simulink model "VSCHVDCunitblackstart"  (R2025b)
settings: Solver=VariableStepAuto  StartTime=0  StopTime=25  FixedStep=5e-5  RelTol=1e-3
PreLoadFcn:
  | HVDCParameters;
  | BlackStartMMCParameters;
undefined symbols (not defined in the file): DiscIntNeverNeededParam, FRated, frt, gGFM, grid, Lbase, Lr, Lt, lvrt, mGFM, mpptOmega, mpptWindSpeed, Nm, pmsm, PRated, Rc, rpir, Rr, Rt, time, Tpir, Ts, Vbase, Vdcs0, VRated, Vt2, windController, windTurbine, Zbase
libraries: fl_lib x47, ee_lib x41, nesl_utility x33, eeGeneralControl x13, eeTransforms x12, slpidlib x8, eeSinusoidalMeasurementV2 x4, simulink x2, eeSinusoidalMeasurement x1, eeStairGenerator x1
(part 3 of 5)

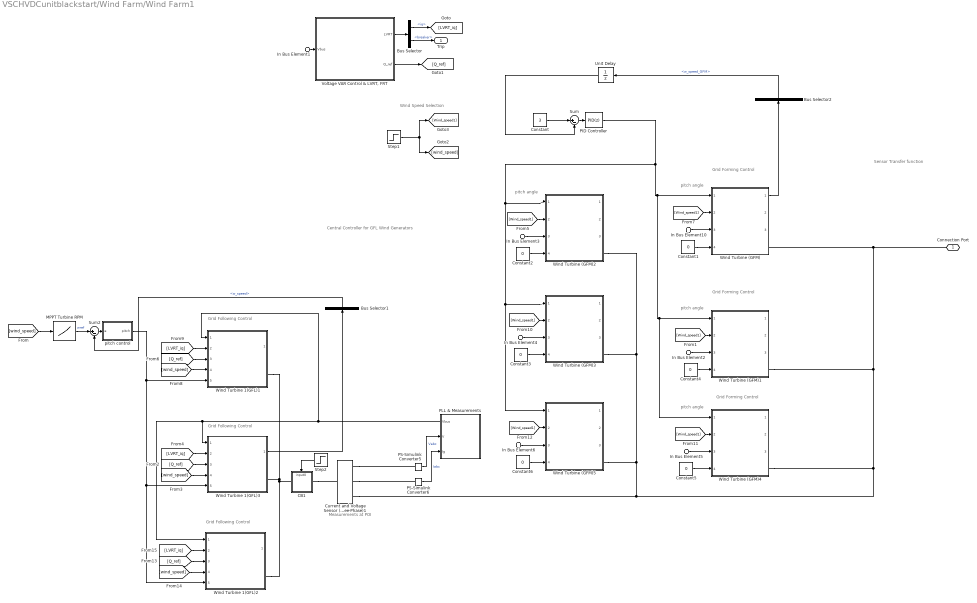
== system VSCHVDCunitblackstart/Wind Farm/Wind Farm1 ==
  note: Central Controller for GFL Wind Generators
  note: Wind Speed Selection
  note: Sensor Transfer function
  note: pitch angle
  note: Grid Forming Control
  note: Grid Forming Control
  note: pitch angle
  note: Grid Forming Control
  note: Measurements at POI
  note: pitch angle
  note: pitch angle
  note: Grid Following Control
  note: Grid Following Control
  note: Grid Following Control
  In Bus Element{1..6,10} (7 alike) : Inport  PortName=us
  Bus Selector : BusSelector  OutputSignals=iq,breaker
  Bus Selector1 : BusSelector  OutputSignals=w_speed
  Bus Selector2 : BusSelector  OutputSignals=w_speed_GFM
  CB1 : Subsystem
      settings: PortSchema="{\"entries\":[{\"content\":{\"sides\":[{\"content\":{\"connectorIds\":[\"LConn1\"]},\"type\":\"ConnectorPlacement.EquallySpacedRectSide\",\"uuid\":\"67c0f727-7c15-41c9-98df-b3c7d57498ed\"},{\"content\":{\"connectorIds\":[\"RConn1\"],\"side\":\"RIGHT\"},\"type\":\"ConnectorPlacement.EquallySpacedRectSide\",\"uuid\":\"7fc39429-ba61-416d-b42b-93e81eb2f426\"},{\"content\":{\"side\":\"TOP\"},\"type\":\"ConnectorPlacement.EquallySpacedRectSide\",\"uuid\":\"c6dd9263-b57a-4cff-a218-af99f2798f29\"},{\"content\":{\"connectorIds\":[\"In1\"],\"side\":\"BOTTOM\"},\"type\":\"ConnectorPlacement.EquallySpacedRectSide\",\"uuid\":\"e2a2ba44-d59d-4e27-adf1-3f94e828ca78\"}]},\"type\":\"ConnectorPlacement.EquallySpacedConnector\",\"uuid\":\"b349a99b-c902-4df9-9c99-34841afb28dd\"}],\"packageUris\":[\"http://schema.mathworks.com/mf0/Connector/R2020b\"],\"version\":\"1.0\"}"
  Constant : Constant  Value=3
  Constant{1..6} (6 alike) : Constant  Value=0
  Current and Voltage Sensor (Three-Phase)1 : ee_lib/Sensors & Transducers/Current and Voltage Sensor (Three-Phase)  vMeasurementType=ee.enum.vmeasurement.lg  outputUnit=ee.enum.unit.pu  SRated=base.mVA A*V  VRated=base.kV V  I_specify=off  I_priority=None  I=[0, 0, 0] A  I_nominal_specify=off  I_nominal_value=1  I_nominal_unit=A  V_specify=off  V_priority=None  V=[0, 0, 0] V  V_nominal_specify=off  V_nominal_value=1  V_nominal_unit=V
      settings: InternalSimscapePortConfiguration="{\"Bottom\":[],\"Left\":[{\"id\":\"N1\",\"label\":\"~1\",\"type\":\"foundation.electrical.three_phase\"}],\"Right\":[{\"id\":\"V_output\",\"label\":\"V\",\"type\":\"output\"},{\"id\":\"I_output\",\"label\":\"I\",\"type\":\"output\"},{\"id\":\"N2\",\"label\":\"~2\",\"type\":\"foundation.electrical.three_phase\"}],\"Top\":[]}"
  MPPT Turbine RPM : Lookup_n-D  NumberOfTableDimensions=1  BreakpointsForDimension1=mpptWindSpeed  Table=mpptOmega  InternalRulePriority=Speed  RndMeth=Simplest
  PID Controller : slpidlib/PID Controller  Controller=PID  Form=Parallel  TimeDomain=Discrete-time  UseExternalTs=off  SampleTime=-1  IntegratorMethod=Forward Euler  FilterMethod=Forward Euler  ControllerParametersSource=internal  P=-0.5  I=-1  UseKiTs=off  D=0  UseExternalDerivativeSource=off  N=100  UseFilter=on  TunerSelectOption=Transfer Function Based (PID Tuner App)  InitialConditionSource=internal  InitialConditionForIntegrator=0  InitialConditionForFilter=0  DifferentiatorICPrevScaledInput=0  ExternalReset=none  TrackingMode=off  Kt=1  LimitOutput=off  SatLimitsSource=internal  UpperSaturationLimit=20  LowerSaturationLimit=-20  LinearizeAsGain=on  AntiWindupMode=back-calculation  Kb=1  LimitIntegrator=off  UpperIntegratorSaturationLimit=inf  LowerIntegratorSaturationLimit=-inf  POutMin=[]  POutMax=[]  IOutMin=[]  IOutMax=[]  DOutMin=[]  DOutMax=[]  NOutMin=[]  NOutMax=[]  SumOutMin=[]  SumOutMax=[]  SaturationOutMin=[]  SaturationOutMax=[]  PParamMin=[]  PParamMax=[]  IParamMin=[]  IParamMax=[]  DParamMin=[]  DParamMax=[]  NParamMin=[]  NParamMax=[]  KbParamMin=[]  KbParamMax=[]  KtParamMin=[]  KtParamMax=[]  KbOutMin=[]  KbOutMax=[]  KtOutMin=[]  KtOutMax=[]  IntegratorOutMin=[]  IntegratorOutMax=[]  FilterOutMin=[]  FilterOutMax=[]  SumI1OutMin=[]  SumI1OutMax=[]  SumI2OutMin=[]  SumI2OutMax=[]  SumI3OutMin=[]  SumI3OutMax=[]  SumI4OutMin=[]  SumI4OutMax=[]  SumDOutMin=[]  SumDOutMax=[]  DifferentiatorOutMin=[]  DifferentiatorOutMax=[]  FilterDiffOutCoefMin=[]  FilterDiffOutCoefMax=[]  ReciprocalOutMin=[]  ReciprocalOutMax=[]  SumDenOutMin=[]  SumDenOutMax=[]  SumNumOutMin=[]  SumNumOutMax=[]  DivideOutMin=[]  DivideOutMax=[]  UdiffTsProdOutMin=[]  UdiffTsProdOutMax=[]  NTsProdOutMin=[]  NTsProdOutMax=[]  UintegralTsProdOutMin=[]  UintegralTsProdOutMax=[]  UngainTsProdOutMin=[]  UngainTsProdOutMax=[]  ClampingZeroOutDataTypeStr=Inherit: Inherit via back propagation  ClampingZeroOutMin=[]  ClampingZeroOutMax=[]  FilterDenConstantOutDataTypeStr=Inherit: Inherit via back propagation  FilterDenConstantOutMin=[]  FilterDenConstantOutMax=[]  PCopyOutDataTypeStr=Inherit: Inherit via back propagation  PCopyOutMin=[]  PCopyOutMax=[]  NCopyOutDataTypeStr=Inherit: Inherit via back propagation  NCopyOutMin=[]  NCopyOutMax=[]  IntegratorContinuousStateAttributes=''  IntegratorStateMustResolveToSignalObject=off  IntegratorRTWStateStorageClass=Auto  FilterContinuousStateAttributes=''  FilterStateMustResolveToSignalObject=off  FilterRTWStateStorageClass=Auto  ParallelPVariant=InternalParameters  IdealPVariant=Disabled  IVariant=InternalParameters  DVariant=InternalParameters  IntegratorVariant=Discrete  SatVariant=Disabled  AWVariant=Passthrough  PCopyVariant=Disabled  TRVariant=Disabled  FdbkBlocksVariant=Forward  IdealPFdbkVariant=Disabled  SatFdbkVariant=Disabled  DerivativeFilterVariant=ForwardEulerFilter  NVariant=InternalParameters  NCopyVariant=Disabled  FilterICVariant=InternalICsFilter  IntegratorICVariant=InternalICs  ExternalResetVariant=Disabled  TRSumVariant=Passthrough  SumFdbkVariant=Disabled  SumVariant=Sum_PID  TsampFilterVariant=InternalTs  TsampNgainVariant=Passthrough  TsampIntegralVariant=Disabled_SignalSpec  ExternalSaturationOutDataTypeStr=Inherit: Same as second input  DerivativeSourceVariant=ErrorSignal  PreIntVariant=InternalPreInt
  PLL & Measurements : Subsystem
      settings: PortSchema="{\"entries\":[{\"content\":{\"sides\":[{\"content\":{\"connectorIds\":[\"Out1\",\"In1\",\"In2\"]},\"type\":\"ConnectorPlacement.EquallySpacedRectSide\",\"uuid\":\"76485780-20fe-4fcf-8224-69648da6ed2a\"},{\"content\":{\"side\":\"RIGHT\"},\"type\":\"ConnectorPlacement.EquallySpacedRectSide\",\"uuid\":\"f19a6390-e634-42c7-8d46-4cd80cbab182\"},{\"content\":{\"side\":\"TOP\"},\"type\":\"ConnectorPlacement.EquallySpacedRectSide\",\"uuid\":\"87682f72-1844-428e-be70-ad7ca3191ee3\"}]},\"type\":\"ConnectorPlacement.EquallySpacedConnector\",\"uuid\":\"f2136b07-48ec-402b-adb3-18c0bac2157c\"}],\"packageUris\":[\"http://schema.mathworks.com/mf0/Connector/R2020b\"],\"version\":\"1.0\"}"
      mask Display: image('measurements.png'); % Use "Edit Image" on toolstrip to change.
  PS-Simulink Converter5 : nesl_utility/PS-Simulink Converter  PhysicalDomain=network_engine_domain  SubClassName=ps_output  LeftPortType=input  RightPortType=output  PseudoPeriodic=off  Frequencies=[]  VectorFormat=inherit  Unit=inherit  AffineConversion=off
  PS-Simulink Converter6 : nesl_utility/PS-Simulink Converter  PhysicalDomain=network_engine_domain  SubClassName=ps_output  LeftPortType=input  RightPortType=output  PseudoPeriodic=off  Frequencies=[]  VectorFormat=inherit  Unit=inherit  AffineConversion=off
  Step1 : Step  Time=time.wind  Before=11  After=11  SampleTime=5e-5  ZeroCross=off
  Step2 : Step  Time=6  Before=1  After=0  SampleTime=Ts
  Sum : Sum  Inputs=|+-
  Sum2 : Sum  Inputs=|+-
  Unit Delay : UnitDelay  SampleTime=-1  HasFrameUpgradeWarning=on
  "Voltage VAR Control & LVRT, FRT" : Subsystem
      mask Display: image('LVRT_4.png');
  Wind Turbine (GFM){,1..5} (6 alike) : Subsystem  ReferencedSubsystem=gfmWind  Control=VSM Using Turbine Inertia  V_ref=gGFM.vref  Q_ref=gGFM.qref  Kq=gGFM.kq  Kt=gGFM.kt  KqI=mGFM.kq  Kp=mGFM.kp*10  Kd=gGFM.kd  Kj=gGFM.kj  H=mGFM.h  D=mGFM.d  Vd_ref=mGFM.Vd  frequency1=gGFM.fref  frequency=mGFM.fref  Spref=Curtailed Power Operation  tstart=0  Vslope=1  Pstart=1  Pslope=1  x_vir=mGFM.x_vir  x_vir1=gGFM.r_vir  r_vir1=gGFM.x_vir  Imax1=gGFM.Imax  Imax=mGFM.Imax  r_vir=mGFM.r_vir  Kpq_mpp=pmsm.lq*pmsm.alpha  Kpd_mpp=pmsm.ld*pmsm.alpha  Kiq_mpp=pmsm.rs*pmsm.alpha  Kid_mpp=pmsm.rs*pmsm.alpha  Kpq=pmsm.lq*pmsm.alpha  Kpd=pmsm.ld*pmsm.alpha  Kiq=pmsm.rs*pmsm.alpha  Kid=pmsm.rs*pmsm.alpha  Kp_dc_sm=mGFM.kpdc  Ki_dc_sm=mGFM.kidc  wt1=0.01  rt1=0.01  pitch1=windTurbine.pitch  cp1=windTurbine.cp  airDensity1=windTurbine.airDensity  TSR1=windTurbine.TSR  Radius1=windTurbine.turbineRadius  wt=0.01  rt=0.01  pitch=windTurbine.pitch  cp=windTurbine.cp  airDensity=windTurbine.airDensity  Radius=windTurbine.turbineRadius  TSR=windTurbine.TSR  Inertia1=windTurbine.inertia  Inertia=windTurbine.inertia  psim1=pmsm.psim  p1=pmsm.p  Rs1=pmsm.rs  Lq1=pmsm.lq  Ld1=pmsm.ld  Ld=pmsm.ld  Lq=pmsm.lq  Rs=pmsm.rs  p=pmsm.p  psim=pmsm.psim
  Wind Turbine 1(GFL)1 : Subsystem  ReferencedSubsystem=WindGFLMpp  p=pmsm.p  psim=pmsm.psim  Rs=pmsm.rs  Ld=pmsm.ld  Lq=pmsm.lq  Kdip_sm=pmsm.ld*pmsm.alpha  Kdii_sm=pmsm.rs*pmsm.alpha  Kqip_sm=pmsm.lq*pmsm.alpha  Kqii_sm=pmsm.rs*pmsm.alpha  airDensity=windTurbine.airDensity  turbineRadius=windTurbine.turbineRadius  pitch=windTurbine.pitch  TSR=windTurbine.TSR  cp=windTurbine.cp  wt=0.01  rt=0.01  Inertia=windTurbine.inertia/100  Kp_dc=windController.kpv  Ki_dc=windController.kiv  Kdpi_g=windController.kpic  Kdii_g=windController.kiic  Kqpi_g=windController.kpic  Kqii_g=windController.kiic  blk=Enabled  slop=0.8  tst=6
  Wind Turbine 1(GFL)2 : Subsystem  ReferencedSubsystem=WindGFLMpp  p=pmsm.p  psim=pmsm.psim  Rs=pmsm.rs  Ld=pmsm.ld  Lq=pmsm.lq  Kdip_sm=pmsm.ld*pmsm.alpha  Kdii_sm=pmsm.rs*pmsm.alpha  Kqip_sm=pmsm.lq*pmsm.alpha  Kqii_sm=pmsm.rs*pmsm.alpha  airDensity=windTurbine.airDensity  turbineRadius=windTurbine.turbineRadius  pitch=windTurbine.pitch  TSR=windTurbine.TSR  cp=windTurbine.cp  wt=0.01  rt=0.01  Inertia=windTurbine.inertia/100  Kp_dc=windController.kpv  Ki_dc=windController.kiv  Kdpi_g=windController.kpic  Kdii_g=windController.kiic  Kqpi_g=windController.kpic  Kqii_g=windController.kiic  blk=Enabled  slop=0.8  tst=6
  Wind Turbine 1(GFL)3 : Subsystem  ReferencedSubsystem=WindGFLMpp  p=pmsm.p  psim=pmsm.psim  Rs=pmsm.rs  Ld=pmsm.ld  Lq=pmsm.lq  Kdip_sm=pmsm.ld*pmsm.alpha  Kdii_sm=pmsm.rs*pmsm.alpha  Kqip_sm=pmsm.lq*pmsm.alpha  Kqii_sm=pmsm.rs*pmsm.alpha  airDensity=windTurbine.airDensity  turbineRadius=windTurbine.turbineRadius  pitch=windTurbine.pitch  TSR=windTurbine.TSR  cp=windTurbine.cp  wt=0.01  rt=0.01  Inertia=windTurbine.inertia/100  Kp_dc=windController.kpv  Ki_dc=windController.kiv  Kdpi_g=windController.kpic  Kdii_g=windController.kiic  Kqpi_g=windController.kpic  Kqii_g=windController.kiic  blk=Enabled  slop=0.8  tst=6
  pitch control : Subsystem
      mask Display: disp('Pitch Control')
  Connection Port : PMIOPort  Side=Left
  Trip : Outport
  wires:
  "Voltage VAR Control & LVRT, FRT"/1(LVRT) -> Bus Selector/1
  In Bus Element1/1 -> "Voltage VAR Control & LVRT, FRT"/1(Vbus)
  Bus Selector/2 -> Trip/1  "<breaker>"
  "Voltage VAR Control & LVRT, FRT"/2(Q_ref) -> [Q_ref]
  Bus Selector/1 -> [LVRT_iq]  "<iq>"
  Bus Selector2/1 -> Unit Delay/1  "<w_speed_GFM>"
  Wind Turbine (GFM)/1 -> Bus Selector2/1
  Step1/1 -> [Wind_speed1], [wind_speed]
  [Wind_speed1] -> Wind Turbine (GFM)/2
  In Bus Element10/1 -> Wind Turbine (GFM)/3
  Unit Delay/1 -> Sum/2
  Sum/1 -> PID Controller/1
  Constant/1 -> Sum/1
  [Wind_speed1] -> Wind Turbine (GFM)1/2
  In Bus Element2/1 -> Wind Turbine (GFM)1/3
  [LVRT_iq] -> Wind Turbine 1(GFL)3/2
  [Q_ref] -> Wind Turbine 1(GFL)3/3
  [wind_speed] -> Wind Turbine 1(GFL)3/4
  Wind Turbine 1(GFL)3/1 -> Bus Selector1/1
  [wind_speed] -> MPPT Turbine RPM/1
  MPPT Turbine RPM/1 -> Sum2/1  "wref"
  Bus Selector1/1 -> Sum2/2  "<w_speed>"
  Sum2/1 -> pitch control/1(e)
  PS-Simulink Converter5/1 -> PLL & Measurements/1(V)  "Vabc"
  PS-Simulink Converter6/1 -> PLL & Measurements/2(Ig)  "Iabc"
  Step2/1 -> CB1/1(input0)
  In Bus Element3/1 -> Wind Turbine (GFM)2/3
  [Wind_speed1] -> Wind Turbine (GFM)2/2
  [Q_ref] -> Wind Turbine 1(GFL)1/3
  pitch control/1(pitch) -> Wind Turbine 1(GFL)2/5, Wind Turbine 1(GFL)3/5, Wind Turbine 1(GFL)1/5
  [LVRT_iq] -> Wind Turbine 1(GFL)1/2
  [wind_speed] -> Wind Turbine 1(GFL)1/4
  [Wind_speed1] -> Wind Turbine (GFM)3/2
  In Bus Element4/1 -> Wind Turbine (GFM)3/3
  [Wind_speed1] -> Wind Turbine (GFM)4/2
  PID Controller/1 -> Wind Turbine (GFM)4/1, Wind Turbine (GFM)1/1, Wind Turbine (GFM)/1, Wind Turbine (GFM)5/1, Wind Turbine (GFM)3/1, Wind Turbine (GFM)2/1
  In Bus Element6/1 -> Wind Turbine (GFM)5/3
  [Wind_speed1] -> Wind Turbine (GFM)5/2
  In Bus Element5/1 -> Wind Turbine (GFM)4/3
  [LVRT_iq] -> Wind Turbine 1(GFL)2/2
  [Q_ref] -> Wind Turbine 1(GFL)2/3
  PLL & Measurements/1(Vbus) -> Wind Turbine 1(GFL)1/1, Wind Turbine 1(GFL)3/1, Wind Turbine 1(GFL)2/1
  [wind_speed] -> Wind Turbine 1(GFL)2/4
  Constant1/1 -> Wind Turbine (GFM)/4
  Constant2/1 -> Wind Turbine (GFM)2/4
  Constant3/1 -> Wind Turbine (GFM)3/4
  Constant4/1 -> Wind Turbine (GFM)1/4
  Constant5/1 -> Wind Turbine (GFM)4/4
  Constant6/1 -> Wind Turbine (GFM)5/4
  connections:
  Wind Turbine (GFM)1/RConn1 -- Wind Turbine (GFM)2/RConn1 -- Wind Turbine (GFM)3/RConn1 -- Wind Turbine (GFM)5/RConn1 -- Current and Voltage Sensor (Three-Phase)1/RConn3 -- Wind Turbine (GFM)4/RConn1 -- Wind Turbine (GFM)/RConn1 -- Connection Port/RConn1
  Current and Voltage Sensor (Three-Phase)1/RConn1 -- PS-Simulink Converter5/LConn1
  Current and Voltage Sensor (Three-Phase)1/RConn2 -- PS-Simulink Converter6/LConn1
  Wind Turbine 1(GFL)3/RConn1 -- CB1/LConn1 -- Wind Turbine 1(GFL)2/RConn1 -- Wind Turbine 1(GFL)1/RConn1
  CB1/RConn1 -- Current and Voltage Sensor (Three-Phase)1/LConn1

== system VSCHVDCunitblackstart/Control/Sending-end and receiving-end control/Offshore Control ==
  VdcRef : Inport
  Qref : Inport  Port=2
  Vabcg : Inport  Port=3
  Iabcg : Inport  Port=4
  Vdcp : Inport  Port=5
  Vdcn : Inport  Port=6
  Constant : Constant  Value=0
  Control : Subsystem
  Measurements : Subsystem
  S : Outport
  wires:
  Control/1(S) -> S/1
  Vdcn/1 -> Measurements/4(Vdcn)
  Vdcp/1 -> Measurements/3(Vdcp)
  Iabcg/1 -> Measurements/2(Iabcg)
  Vabcg/1 -> Measurements/1(Vabcg)
  Qref/1 -> Control/2(Qref)  "Qref"
  Measurements/1(omega) -> Control/3(omega)
  Measurements/2(theta) -> Control/4(theta)
  Measurements/3(Vdg) -> Control/5(Vd)
  Measurements/4(idg) -> Control/6(idg)
  Measurements/5(iqg) -> Control/7(iqg)
  Measurements/6(VdcpF) -> Control/8(Vdcp)
  Measurements/7(VdcnF) -> Control/9(Vdcn)
  Measurements/8(Qmea) -> Control/10(Qmea)  "Qmea"
  VdcRef/1 -> Control/1(VdcRef)  "VdcRef"
  Constant/1 -> Control/11(Vstart)

== system VSCHVDCunitblackstart/Control/Sending-end and receiving-end control/Onshore Control ==
  note: -0.05
  Vabcg : Inport
  Iabcg : Inport  Port=2
  Vdcp : Inport  Port=3
  Vdcn : Inport  Port=4
  Pref : Inport  Port=5
  Pm : Inport  Port=6
  Qref : Inport  Port=7
  Qm : Inport  Port=8
  Vref : Inport  Port=9
  Constant1 : Constant  Value=0
  Control : Subsystem
  Gain : Gain  Gain=Kq
  Measurements : Subsystem
  Sum : Sum  Inputs=|+-
  Sum1 : Sum  Inputs=|++
  Unit Delay : UnitDelay  SampleTime=-1  HasFrameUpgradeWarning=on
  S : Outport
  wires:
  Constant1/1 -> Control/2(Vqref)  "Vqref"
  Measurements/1(VdcpF) -> Control/3(Vdcp)
  Measurements/2(VdcnF) -> Control/4(Vdcn)
  Vabcg/1 -> Measurements/1(Vabcg)
  Iabcg/1 -> Measurements/2(Iabcg)
  Vdcp/1 -> Measurements/3(Vdcp)
  Vdcn/1 -> Measurements/4(Vdcn)
  Control/1(S) -> S/1
  Measurements/5(theta) -> Control/7(theta)
  Measurements/3(Vdg) -> Control/5(Vdmea)
  Measurements/4(Vqg) -> Control/6(Vqmea)
  Pref/1 -> Measurements/5(Pref)  "Pref"
  Qm/1 -> Unit Delay/1  "Qmea"
  Unit Delay/1 -> Sum/2
  Vref/1 -> Sum1/1  "Vd"
  Sum/1 -> Gain/1
  Gain/1 -> Sum1/2
  Sum1/1 -> Control/1(Vdref)  "Vref"
  Qref/1 -> Sum/1  "Qref"
  Pm/1 -> Measurements/6(Pm)  "Pmea"

== system VSCHVDCunitblackstart/Onshore Grid/CB1/Subsystem1 ==
  input0 : Inport
  Gain : Gain  Gain=1e9
  PS Gain : fl_lib/Physical Signals/Functions/PS Gain  gain=5e-4
  Phase Splitter : ee_lib/Connectors & References/Phase Splitter
  Phase Splitter1 : ee_lib/Connectors & References/Phase Splitter
  Simulink-PS Converter : nesl_utility/Simulink-PS Converter  PhysicalDomain=network_engine_domain  SubClassName=ps_input  LeftPortType=input  RightPortType=output  PseudoPeriodic=off  Frequencies=[]  NoiseDistribution=none  NoiseParameters=[]  Unit=1  AffineConversion=off  FilteringAndDerivatives=provide  SimscapeFilterOrder=1  InputFilterTimeConstant=0.001  UdotUserProvided=0
  Variable Inductor : ee_lib/Passive/Variable Inductor  prm=2  Lmin=1e-6 H  g=1e-10 1/Ohm  i0=0 A  phi0=0 Wb
      settings: InternalSimscapePortConfiguration="{\"Bottom\":[],\"Left\":[{\"id\":\"L\",\"label\":\"L\",\"type\":\"input\"},{\"id\":\"p\",\"label\":\"+\",\"type\":\"foundation.electrical.electrical\"}],\"Right\":[{\"id\":\"n\",\"label\":\"-\",\"type\":\"foundation.electrical.electrical\"}],\"Top\":[]}"
  Variable Inductor1 : ee_lib/Passive/Variable Inductor  prm=2  Lmin=1e-6 H  g=1e-10 1/Ohm  i0=0 A  phi0=0 Wb
      settings: InternalSimscapePortConfiguration="{\"Bottom\":[],\"Left\":[{\"id\":\"L\",\"label\":\"L\",\"type\":\"input\"},{\"id\":\"p\",\"label\":\"+\",\"type\":\"foundation.electrical.electrical\"}],\"Right\":[{\"id\":\"n\",\"label\":\"-\",\"type\":\"foundation.electrical.electrical\"}],\"Top\":[]}"
  Variable Inductor2 : ee_lib/Passive/Variable Inductor  prm=2  Lmin=1e-6 H  g=1e-10 1/Ohm  i0=0 A  phi0=0 Wb
      settings: InternalSimscapePortConfiguration="{\"Bottom\":[],\"Left\":[{\"id\":\"L\",\"label\":\"L\",\"type\":\"input\"},{\"id\":\"p\",\"label\":\"+\",\"type\":\"foundation.electrical.electrical\"}],\"Right\":[{\"id\":\"n\",\"label\":\"-\",\"type\":\"foundation.electrical.electrical\"}],\"Top\":[]}"
  Variable Resistor : fl_lib/Electrical/Electrical Elements/Variable Resistor  Rmin=1e-4 Ohm  thermalEnable=false  thermal_mass=1 J/K  i_specify=off  i_priority=None  i=0 A  i_nominal_specify=off  i_nominal_value=1  i_nominal_unit=A  v_specify=off  v_priority=None  v=0 V  v_nominal_specify=off  v_nominal_value=1  v_nominal_unit=V  T_specify=off  T_priority=None  T=300 K  T_nominal_specify=off  T_nominal_value=1  T_nominal_unit=K
  Variable Resistor1 : fl_lib/Electrical/Electrical Elements/Variable Resistor  Rmin=1e-4 Ohm  thermalEnable=false  thermal_mass=1 J/K  i_specify=off  i_priority=None  i=0 A  i_nominal_specify=off  i_nominal_value=1  i_nominal_unit=A  v_specify=off  v_priority=None  v=0 V  v_nominal_specify=off  v_nominal_value=1  v_nominal_unit=V  T_specify=off  T_priority=None  T=300 K  T_nominal_specify=off  T_nominal_value=1  T_nominal_unit=K
  Variable Resistor2 : fl_lib/Electrical/Electrical Elements/Variable Resistor  Rmin=1e-4 Ohm  thermalEnable=false  thermal_mass=1 J/K  i_specify=off  i_priority=None  i=0 A  i_nominal_specify=off  i_nominal_value=1  i_nominal_unit=A  v_specify=off  v_priority=None  v=0 V  v_nominal_specify=off  v_nominal_value=1  v_nominal_unit=V  T_specify=off  T_priority=None  T=300 K  T_nominal_specify=off  T_nominal_value=1  T_nominal_unit=K
  Conn1 : PMIOPort  Side=Left
  Conn2 : PMIOPort  Port=2  Side=Right
  wires:
  input0/1 -> Gain/1
  Gain/1 -> Simulink-PS Converter/1
  connections:
  Variable Inductor2/LConn2 -- Variable Resistor2/RConn1
  Phase Splitter1/RConn3 -- Variable Inductor2/RConn1
  Variable Inductor2/LConn1 -- PS Gain/RConn1 -- Variable Inductor/LConn1 -- Variable Inductor1/LConn1
  Phase Splitter1/RConn2 -- Variable Inductor1/RConn1
  Phase Splitter1/RConn1 -- Variable Inductor/RConn1
  Simulink-PS Converter/RConn1 -- PS Gain/LConn1 -- Variable Resistor2/LConn1 -- Variable Resistor1/LConn1 -- Variable Resistor/LConn1
  Variable Inductor/LConn2 -- Variable Resistor/RConn1
  Phase Splitter/LConn1 -- Conn2/RConn1
  Phase Splitter/RConn1 -- Variable Resistor/LConn2
  Phase Splitter/RConn2 -- Variable Resistor1/LConn2
  Phase Splitter/RConn3 -- Variable Resistor2/LConn2
  Phase Splitter1/LConn1 -- Conn1/RConn1
  Variable Inductor1/LConn2 -- Variable Resistor1/RConn1

== system VSCHVDCunitblackstart/Onshore Grid/CB2/Subsystem1 ==
  input0 : Inport
  Gain : Gain  Gain=1e9
  PS Gain : fl_lib/Physical Signals/Functions/PS Gain  gain=5e-4
  Phase Splitter : ee_lib/Connectors & References/Phase Splitter
  Phase Splitter1 : ee_lib/Connectors & References/Phase Splitter
  Simulink-PS Converter : nesl_utility/Simulink-PS Converter  PhysicalDomain=network_engine_domain  SubClassName=ps_input  LeftPortType=input  RightPortType=output  PseudoPeriodic=off  Frequencies=[]  NoiseDistribution=none  NoiseParameters=[]  Unit=1  AffineConversion=off  FilteringAndDerivatives=provide  SimscapeFilterOrder=1  InputFilterTimeConstant=0.001  UdotUserProvided=0
  Variable Inductor : ee_lib/Passive/Variable Inductor  prm=2  Lmin=1e-6 H  g=1e-10 1/Ohm  i0=0 A  phi0=0 Wb
      settings: InternalSimscapePortConfiguration="{\"Bottom\":[],\"Left\":[{\"id\":\"L\",\"label\":\"L\",\"type\":\"input\"},{\"id\":\"p\",\"label\":\"+\",\"type\":\"foundation.electrical.electrical\"}],\"Right\":[{\"id\":\"n\",\"label\":\"-\",\"type\":\"foundation.electrical.electrical\"}],\"Top\":[]}"
  Variable Inductor1 : ee_lib/Passive/Variable Inductor  prm=2  Lmin=1e-6 H  g=1e-10 1/Ohm  i0=0 A  phi0=0 Wb
      settings: InternalSimscapePortConfiguration="{\"Bottom\":[],\"Left\":[{\"id\":\"L\",\"label\":\"L\",\"type\":\"input\"},{\"id\":\"p\",\"label\":\"+\",\"type\":\"foundation.electrical.electrical\"}],\"Right\":[{\"id\":\"n\",\"label\":\"-\",\"type\":\"foundation.electrical.electrical\"}],\"Top\":[]}"
  Variable Inductor2 : ee_lib/Passive/Variable Inductor  prm=2  Lmin=1e-6 H  g=1e-10 1/Ohm  i0=0 A  phi0=0 Wb
      settings: InternalSimscapePortConfiguration="{\"Bottom\":[],\"Left\":[{\"id\":\"L\",\"label\":\"L\",\"type\":\"input\"},{\"id\":\"p\",\"label\":\"+\",\"type\":\"foundation.electrical.electrical\"}],\"Right\":[{\"id\":\"n\",\"label\":\"-\",\"type\":\"foundation.electrical.electrical\"}],\"Top\":[]}"
  Variable Resistor : fl_lib/Electrical/Electrical Elements/Variable Resistor  Rmin=1e-4 Ohm  thermalEnable=false  thermal_mass=1 J/K  i_specify=off  i_priority=None  i=0 A  i_nominal_specify=off  i_nominal_value=1  i_nominal_unit=A  v_specify=off  v_priority=None  v=0 V  v_nominal_specify=off  v_nominal_value=1  v_nominal_unit=V  T_specify=off  T_priority=None  T=300 K  T_nominal_specify=off  T_nominal_value=1  T_nominal_unit=K
  Variable Resistor1 : fl_lib/Electrical/Electrical Elements/Variable Resistor  Rmin=1e-4 Ohm  thermalEnable=false  thermal_mass=1 J/K  i_specify=off  i_priority=None  i=0 A  i_nominal_specify=off  i_nominal_value=1  i_nominal_unit=A  v_specify=off  v_priority=None  v=0 V  v_nominal_specify=off  v_nominal_value=1  v_nominal_unit=V  T_specify=off  T_priority=None  T=300 K  T_nominal_specify=off  T_nominal_value=1  T_nominal_unit=K
  Variable Resistor2 : fl_lib/Electrical/Electrical Elements/Variable Resistor  Rmin=1e-4 Ohm  thermalEnable=false  thermal_mass=1 J/K  i_specify=off  i_priority=None  i=0 A  i_nominal_specify=off  i_nominal_value=1  i_nominal_unit=A  v_specify=off  v_priority=None  v=0 V  v_nominal_specify=off  v_nominal_value=1  v_nominal_unit=V  T_specify=off  T_priority=None  T=300 K  T_nominal_specify=off  T_nominal_value=1  T_nominal_unit=K
  Conn1 : PMIOPort  Side=Left
  Conn2 : PMIOPort  Port=2  Side=Right
  wires:
  input0/1 -> Gain/1
  Gain/1 -> Simulink-PS Converter/1
  connections:
  Variable Inductor2/LConn2 -- Variable Resistor2/RConn1
  Phase Splitter1/RConn3 -- Variable Inductor2/RConn1
  Variable Inductor2/LConn1 -- PS Gain/RConn1 -- Variable Inductor/LConn1 -- Variable Inductor1/LConn1
  Phase Splitter1/RConn2 -- Variable Inductor1/RConn1
  Phase Splitter1/RConn1 -- Variable Inductor/RConn1
  Simulink-PS Converter/RConn1 -- PS Gain/LConn1 -- Variable Resistor2/LConn1 -- Variable Resistor1/LConn1 -- Variable Resistor/LConn1
  Variable Inductor/LConn2 -- Variable Resistor/RConn1
  Phase Splitter/LConn1 -- Conn2/RConn1
  Phase Splitter/RConn1 -- Variable Resistor/LConn2
  Phase Splitter/RConn2 -- Variable Resistor1/LConn2
  Phase Splitter/RConn3 -- Variable Resistor2/LConn2
  Phase Splitter1/LConn1 -- Conn1/RConn1
  Variable Inductor1/LConn2 -- Variable Resistor1/RConn1

== system VSCHVDCunitblackstart/Onshore Grid/PLL & Measurements/Measurement2 ==
  u : Inport
  Vg : Outport
  wires:
  u/1 -> Vg/1

== system VSCHVDCunitblackstart/Onshore Grid/PLL & Measurements/PLL ==
  abc : Inport
  "Sinusoidal Measurement (PLL, Three-Phase)1" : eeSinusoidalMeasurementV2/Sinusoidal Measurement (PLL, Three-Phase)  InputFilter=on  InputNormalization=off  Kp_LF=pll.kp  Ki_LF=pll.ki  F0=grid.frequency  Theta0=0  Ts=Ts
      settings: LibrarySourceBlock=|
      | ee_sl_lib/Measurements/Sinusoidal Measurement
      | (PLL, Three-Phase)
  mag : Outport
  freq : Outport  Port=2
  angle : Outport  Port=3
  wires:
  "Sinusoidal Measurement (PLL, Three-Phase)1"/3 -> mag/1
  "Sinusoidal Measurement (PLL, Three-Phase)1"/2 -> angle/1
  abc/1 -> "Sinusoidal Measurement (PLL, Three-Phase)1"/1
  "Sinusoidal Measurement (PLL, Three-Phase)1"/1 -> freq/1

== system VSCHVDCunitblackstart/Wind Farm/CB1/Subsystem1 ==
  input0 : Inport
  Gain : Gain  Gain=1e9
  Phase Splitter : ee_lib/Connectors & References/Phase Splitter
  Phase Splitter1 : ee_lib/Connectors & References/Phase Splitter
  Simulink-PS Converter : nesl_utility/Simulink-PS Converter  PhysicalDomain=network_engine_domain  SubClassName=ps_input  LeftPortType=input  RightPortType=output  PseudoPeriodic=off  Frequencies=[]  NoiseDistribution=none  NoiseParameters=[]  Unit=1  AffineConversion=off  FilteringAndDerivatives=provide  SimscapeFilterOrder=1  InputFilterTimeConstant=0.001  UdotUserProvided=0
  Variable Resistor : fl_lib/Electrical/Electrical Elements/Variable Resistor  Rmin=1e-4 Ohm  thermalEnable=false  thermal_mass=1 J/K  i_specify=off  i_priority=None  i=0 A  i_nominal_specify=off  i_nominal_value=1  i_nominal_unit=A  v_specify=off  v_priority=None  v=0 V  v_nominal_specify=off  v_nominal_value=1  v_nominal_unit=V  T_specify=off  T_priority=None  T=300 K  T_nominal_specify=off  T_nominal_value=1  T_nominal_unit=K
  Variable Resistor1 : fl_lib/Electrical/Electrical Elements/Variable Resistor  Rmin=1e-4 Ohm  thermalEnable=false  thermal_mass=1 J/K  i_specify=off  i_priority=None  i=0 A  i_nominal_specify=off  i_nominal_value=1  i_nominal_unit=A  v_specify=off  v_priority=None  v=0 V  v_nominal_specify=off  v_nominal_value=1  v_nominal_unit=V  T_specify=off  T_priority=None  T=300 K  T_nominal_specify=off  T_nominal_value=1  T_nominal_unit=K
  Variable Resistor2 : fl_lib/Electrical/Electrical Elements/Variable Resistor  Rmin=1e-4 Ohm  thermalEnable=false  thermal_mass=1 J/K  i_specify=off  i_priority=None  i=0 A  i_nominal_specify=off  i_nominal_value=1  i_nominal_unit=A  v_specify=off  v_priority=None  v=0 V  v_nominal_specify=off  v_nominal_value=1  v_nominal_unit=V  T_specify=off  T_priority=None  T=300 K  T_nominal_specify=off  T_nominal_value=1  T_nominal_unit=K
  Conn1 : PMIOPort  Side=Left
  Conn2 : PMIOPort  Port=2  Side=Right
  wires:
  input0/1 -> Gain/1
  Gain/1 -> Simulink-PS Converter/1
  connections:
  Simulink-PS Converter/RConn1 -- Variable Resistor2/LConn1 -- Variable Resistor1/LConn1 -- Variable Resistor/LConn1
  Phase Splitter/LConn1 -- Conn2/RConn1
  Phase Splitter/RConn1 -- Variable Resistor/LConn2
  Phase Splitter/RConn2 -- Variable Resistor1/LConn2
  Phase Splitter/RConn3 -- Variable Resistor2/LConn2
  Phase Splitter1/LConn1 -- Conn1/RConn1
  Variable Resistor/RConn1 -- Phase Splitter1/RConn1
  Phase Splitter1/RConn2 -- Variable Resistor1/RConn1
  Variable Resistor2/RConn1 -- Phase Splitter1/RConn3

== system VSCHVDCunitblackstart/Wind Farm/CB2/Subsystem1 ==
  input0 : Inport
  Gain : Gain  Gain=1e9
  Phase Splitter : ee_lib/Connectors & References/Phase Splitter
  Phase Splitter1 : ee_lib/Connectors & References/Phase Splitter
  Simulink-PS Converter : nesl_utility/Simulink-PS Converter  PhysicalDomain=network_engine_domain  SubClassName=ps_input  LeftPortType=input  RightPortType=output  PseudoPeriodic=off  Frequencies=[]  NoiseDistribution=none  NoiseParameters=[]  Unit=1  AffineConversion=off  FilteringAndDerivatives=provide  SimscapeFilterOrder=1  InputFilterTimeConstant=0.001  UdotUserProvided=0
  Variable Resistor : fl_lib/Electrical/Electrical Elements/Variable Resistor  Rmin=1e-4 Ohm  thermalEnable=false  thermal_mass=1 J/K  i_specify=off  i_priority=None  i=0 A  i_nominal_specify=off  i_nominal_value=1  i_nominal_unit=A  v_specify=off  v_priority=None  v=0 V  v_nominal_specify=off  v_nominal_value=1  v_nominal_unit=V  T_specify=off  T_priority=None  T=300 K  T_nominal_specify=off  T_nominal_value=1  T_nominal_unit=K
  Variable Resistor1 : fl_lib/Electrical/Electrical Elements/Variable Resistor  Rmin=1e-4 Ohm  thermalEnable=false  thermal_mass=1 J/K  i_specify=off  i_priority=None  i=0 A  i_nominal_specify=off  i_nominal_value=1  i_nominal_unit=A  v_specify=off  v_priority=None  v=0 V  v_nominal_specify=off  v_nominal_value=1  v_nominal_unit=V  T_specify=off  T_priority=None  T=300 K  T_nominal_specify=off  T_nominal_value=1  T_nominal_unit=K
  Variable Resistor2 : fl_lib/Electrical/Electrical Elements/Variable Resistor  Rmin=1e-4 Ohm  thermalEnable=false  thermal_mass=1 J/K  i_specify=off  i_priority=None  i=0 A  i_nominal_specify=off  i_nominal_value=1  i_nominal_unit=A  v_specify=off  v_priority=None  v=0 V  v_nominal_specify=off  v_nominal_value=1  v_nominal_unit=V  T_specify=off  T_priority=None  T=300 K  T_nominal_specify=off  T_nominal_value=1  T_nominal_unit=K
  Conn1 : PMIOPort  Side=Left
  Conn2 : PMIOPort  Port=2  Side=Right
  wires:
  input0/1 -> Gain/1
  Gain/1 -> Simulink-PS Converter/1
  connections:
  Simulink-PS Converter/RConn1 -- Variable Resistor2/LConn1 -- Variable Resistor1/LConn1 -- Variable Resistor/LConn1
  Phase Splitter/LConn1 -- Conn2/RConn1
  Phase Splitter/RConn1 -- Variable Resistor/LConn2
  Phase Splitter/RConn2 -- Variable Resistor1/LConn2
  Phase Splitter/RConn3 -- Variable Resistor2/LConn2
  Phase Splitter1/LConn1 -- Conn1/RConn1
  Variable Resistor/RConn1 -- Phase Splitter1/RConn1
  Phase Splitter1/RConn2 -- Variable Resistor1/RConn1
  Variable Resistor2/RConn1 -- Phase Splitter1/RConn3

== system VSCHVDCunitblackstart/Wind Farm/CB3/Subsystem1 ==
  input0 : Inport
  Gain : Gain  Gain=1e9
  Phase Splitter : ee_lib/Connectors & References/Phase Splitter
  Phase Splitter1 : ee_lib/Connectors & References/Phase Splitter
  Simulink-PS Converter : nesl_utility/Simulink-PS Converter  PhysicalDomain=network_engine_domain  SubClassName=ps_input  LeftPortType=input  RightPortType=output  PseudoPeriodic=off  Frequencies=[]  NoiseDistribution=none  NoiseParameters=[]  Unit=1  AffineConversion=off  FilteringAndDerivatives=provide  SimscapeFilterOrder=1  InputFilterTimeConstant=0.001  UdotUserProvided=0
  Variable Resistor : fl_lib/Electrical/Electrical Elements/Variable Resistor  Rmin=1e-4 Ohm  thermalEnable=false  thermal_mass=1 J/K  i_specify=off  i_priority=None  i=0 A  i_nominal_specify=off  i_nominal_value=1  i_nominal_unit=A  v_specify=off  v_priority=None  v=0 V  v_nominal_specify=off  v_nominal_value=1  v_nominal_unit=V  T_specify=off  T_priority=None  T=300 K  T_nominal_specify=off  T_nominal_value=1  T_nominal_unit=K
  Variable Resistor1 : fl_lib/Electrical/Electrical Elements/Variable Resistor  Rmin=1e-4 Ohm  thermalEnable=false  thermal_mass=1 J/K  i_specify=off  i_priority=None  i=0 A  i_nominal_specify=off  i_nominal_value=1  i_nominal_unit=A  v_specify=off  v_priority=None  v=0 V  v_nominal_specify=off  v_nominal_value=1  v_nominal_unit=V  T_specify=off  T_priority=None  T=300 K  T_nominal_specify=off  T_nominal_value=1  T_nominal_unit=K
  Variable Resistor2 : fl_lib/Electrical/Electrical Elements/Variable Resistor  Rmin=1e-4 Ohm  thermalEnable=false  thermal_mass=1 J/K  i_specify=off  i_priority=None  i=0 A  i_nominal_specify=off  i_nominal_value=1  i_nominal_unit=A  v_specify=off  v_priority=None  v=0 V  v_nominal_specify=off  v_nominal_value=1  v_nominal_unit=V  T_specify=off  T_priority=None  T=300 K  T_nominal_specify=off  T_nominal_value=1  T_nominal_unit=K
  Conn1 : PMIOPort  Side=Left
  Conn2 : PMIOPort  Port=2  Side=Right
  wires:
  input0/1 -> Gain/1
  Gain/1 -> Simulink-PS Converter/1
  connections:
  Simulink-PS Converter/RConn1 -- Variable Resistor2/LConn1 -- Variable Resistor1/LConn1 -- Variable Resistor/LConn1
  Phase Splitter/LConn1 -- Conn2/RConn1
  Phase Splitter/RConn1 -- Variable Resistor/LConn2
  Phase Splitter/RConn2 -- Variable Resistor1/LConn2
  Phase Splitter/RConn3 -- Variable Resistor2/LConn2
  Phase Splitter1/LConn1 -- Conn1/RConn1
  Variable Resistor/RConn1 -- Phase Splitter1/RConn1
  Phase Splitter1/RConn2 -- Variable Resistor1/RConn1
  Variable Resistor2/RConn1 -- Phase Splitter1/RConn3

== system VSCHVDCunitblackstart/Wind Farm/PLL & Measurements/Measurement1 ==
  u : Inport
  Ig : Outport
  wires:
  u/1 -> Ig/1

== system VSCHVDCunitblackstart/Wind Farm/PLL & Measurements/Measurement2 ==
  u : Inport
  Vg : Outport
  wires:
  u/1 -> Vg/1

== system VSCHVDCunitblackstart/Wind Farm/PLL & Measurements/PLL ==
  abc : Inport
  Ig : Inport  Port=2
  Demux : Demux  Outputs=3
  Demux1 : Demux  Outputs=3
  Park Transform : eeTransforms/Park Transform  AxisAlignment=Q-axis  PowerInvariant=off
  Park Transform1 : eeTransforms/Park Transform  AxisAlignment=Q-axis  PowerInvariant=off
  "Sinusoidal Measurement (PLL, Three-Phase)1" : eeSinusoidalMeasurementV2/Sinusoidal Measurement (PLL, Three-Phase)  InputFilter=on  InputNormalization=off  Kp_LF=pll.kp  Ki_LF=pll.ki  F0=grid.frequency  Theta0=0  Ts=Ts
      settings: LibrarySourceBlock=|
      | ee_sl_lib/Measurements/Sinusoidal Measurement
      | (PLL, Three-Phase)
  Terminator : Terminator
  Terminator1 : Terminator
  abc1 : InportShadow
  mag : Outport
  freq : Outport  Port=2
  angle : Outport  Port=3
  Vd : Outport  Port=4
  Vq : Outport  Port=5
  Id : Outport  Port=6
  Iq : Outport  Port=7
  wires:
  Demux/3 -> Terminator/1
  Park Transform/1 -> Demux/1
  Demux/1 -> Vd/1
  Demux/2 -> Vq/1
  "Sinusoidal Measurement (PLL, Three-Phase)1"/3 -> mag/1
  "Sinusoidal Measurement (PLL, Three-Phase)1"/2 -> angle/1, Park Transform/2, Park Transform1/2
  Ig/1 -> Park Transform1/1
  Demux1/2 -> Iq/1
  Park Transform1/1 -> Demux1/1
  Demux1/1 -> Id/1
  Demux1/3 -> Terminator1/1
  abc1/1 -> Park Transform/1
  abc/1 -> "Sinusoidal Measurement (PLL, Three-Phase)1"/1
  "Sinusoidal Measurement (PLL, Three-Phase)1"/1 -> freq/1

== system VSCHVDCunitblackstart/Wind Farm/Wind Farm/CB1 ==
  input0 : Inport
  Subsystem1 : Subsystem
      settings: PortSchema="{\"entries\":[{\"content\":{\"sides\":[{\"content\":{\"connectorIds\":[\"LConn1\",\"In1\"]},\"type\":\"ConnectorPlacement.EquallySpacedRectSide\",\"uuid\":\"4d523b2f-3490-490d-9193-0c3e52b1c3a1\"},{\"content\":{\"connectorIds\":[\"RConn1\"],\"side\":\"RIGHT\"},\"type\":\"ConnectorPlacement.EquallySpacedRectSide\",\"uuid\":\"1543a14a-65b5-4637-8d41-6da95a6ca307\"},{\"content\":{\"side\":\"TOP\"},\"type\":\"ConnectorPlacement.EquallySpacedRectSide\",\"uuid\":\"9fff8ee8-4727-466f-977a-681c4f14cc56\"}]},\"type\":\"ConnectorPlacement.EquallySpacedConnector\",\"uuid\":\"a46df766-bf17-4bd6-a8b3-579011040ee9\"}],\"packageUris\":[\"http://schema.mathworks.com/mf0/Connector/R2020b\"],\"version\":\"1.0\"}"
  Conn2 : PMIOPort  Side=Left
  Conn1 : PMIOPort  Port=2  Side=Right
  wires:
  input0/1 -> Subsystem1/1(input0)
  connections:
  Conn2/RConn1 -- Subsystem1/RConn1
  Subsystem1/LConn1 -- Conn1/RConn1

== system VSCHVDCunitblackstart/Wind Farm/Wind Farm/Measurements1 ==
  <w_GFM> : Inport
  <Vdc_GFM> : Inport  Port=2
  <P> : Inport  Port=3
  <Q> : Inport  Port=4
  In5 : Inport  Port=5
  Terminator{,1..4} (5 alike) : Terminator
  wires:
  <P>/1 -> Terminator2/1  "P"
  <w_GFM>/1 -> Terminator/1  "Rotational speed"
  <Q>/1 -> Terminator3/1  "Q"
  <Vdc_GFM>/1 -> Terminator1/1  "Vdc"
  In5/1 -> Terminator4/1  "PWF"

== system VSCHVDCunitblackstart/Wind Farm/Wind Farm/Measurements2 ==
  <w_GFM> : Inport
  <Vdc_GFM> : Inport  Port=2
  T : Inport  Port=3
  <P> : Inport  Port=4
  <Q> : Inport  Port=5
  Terminator{,1..4} (5 alike) : Terminator
  wires:
  <P>/1 -> Terminator2/1  "PGFL"
  <w_GFM>/1 -> Terminator/1  "Rotational speed"
  <Q>/1 -> Terminator3/1  "Q"
  <Vdc_GFM>/1 -> Terminator1/1  "Vdc"
  T/1 -> Terminator4/1  "Torque"

== system VSCHVDCunitblackstart/Wind Farm/Wind Farm/PLL & Measurements ==
  V : Inport
  Ig : Inport  Port=2
  Measurement1 : Subsystem
  Measurement2 : Subsystem
  PLL : Subsystem
  Out Bus Element : Outport  PortName=Vbus  Element=Vq
  Out Bus Element1 : Outport  PortName=Vbus  Element=Vd
  Out Bus Element2 : Outport  PortName=Vbus  Element=w
  Out Bus Element3 : Outport  PortName=Vbus  Element=Theta
  Out Bus Element4 : Outport  PortName=Vbus  Element=Vmag
  Out Bus Element5 : Outport  PortName=Vbus  Element=Id
  Out Bus Element6 : Outport  PortName=Vbus  Element=Iq
  wires:
  V/1 -> Measurement2/1(u)
  PLL/2(freq) -> Out Bus Element2/1
  PLL/5(Vq) -> Out Bus Element/1  "Vq"
  PLL/3(angle) -> Out Bus Element3/1
  PLL/4(Vd) -> Out Bus Element1/1
  Measurement2/1(Vg) -> PLL/1(abc)
  PLL/1(mag) -> Out Bus Element4/1  "Vmag"
  Measurement1/1(Ig) -> PLL/2(Ig)
  Ig/1 -> Measurement1/1(u)
  PLL/7(Iq) -> Out Bus Element6/1  "Iq"
  PLL/6(Id) -> Out Bus Element5/1  "Id"

== system VSCHVDCunitblackstart/Wind Farm/Wind Farm/Voltage VAR Control & LVRT, FRT ==
  In Bus Element : Inport  PortName=Vbus  Element=Vmag
  In Bus Element1 : Inport  PortName=Vbus  Element=w
  Data Type Conversion : DataTypeConversion  RndMeth=Nearest  SaturateOnIntegerOverflow=off
  Delay : Delay  DelayLength=100
  Frequency RideThrough : Subsystem
  LVRT Characterstics : Subsystem
  OR : Logic  Operator=OR  IconShape=distinctive  AllPortsSameDT=off  OutDataTypeStr=boolean
  Unit Delay : UnitDelay  SampleTime=-1  HasFrameUpgradeWarning=on
  V_ref : Constant  Value=windController.vRef  SampleTime=Ts
  Voltage Control : Subsystem
  Out Bus Element : Outport  PortName=LVRT  Element=breaker
  Out Bus Element1 : Outport  PortName=LVRT  Element=iq
  Q_ref : Outport  Port=2
  wires:
  In Bus Element/1 -> LVRT Characterstics/1(Vmag), Voltage Control/1(In1)
  LVRT Characterstics/2(iq) -> Out Bus Element1/1
  V_ref/1 -> Voltage Control/2(In2)
  Voltage Control/1(Out1) -> Delay/1
  OR/1 -> Data Type Conversion/1
  LVRT Characterstics/1(Trip Signal) -> OR/1
  In Bus Element1/1 -> Frequency RideThrough/1(f)
  Data Type Conversion/1 -> Unit Delay/1
  Frequency RideThrough/1(Trip  Signal) -> OR/2
  Unit Delay/1 -> Out Bus Element/1
  Delay/1 -> Q_ref/1

== system VSCHVDCunitblackstart/Wind Farm/Wind Farm/pitch control ==
  e : Inport
  Discrete-Time Integrator : DiscreteIntegrator  SampleTime=-1  LimitOutput=on  LowerSaturationLimit=0  ICPrevOutput=DiscIntNeverNeededParam  ICPrevScaledInput=DiscIntNeverNeededParam
  Gain1 : Gain  Gain=-5
  Gain2 : Gain  Gain=-1
  Saturation1 : Saturate  UpperLimit=inf  LowerLimit=0
  Sum1 : Sum  Inputs=|++
  Unit Delay : UnitDelay  SampleTime=-1  HasFrameUpgradeWarning=on
  pitch : Outport
  wires:
  Discrete-Time Integrator/1 -> Sum1/2
  e/1 -> Gain2/1, Gain1/1
  Saturation1/1 -> pitch/1  "pitch"
  Gain2/1 -> Discrete-Time Integrator/1
  Unit Delay/1 -> Sum1/1
  Gain1/1 -> Unit Delay/1
  Sum1/1 -> Saturation1/1

== system VSCHVDCunitblackstart/Wind Farm/Wind Farm1/CB1 ==
  input0 : Inport
  Subsystem1 : Subsystem
      settings: PortSchema="{\"entries\":[{\"content\":{\"sides\":[{\"content\":{\"connectorIds\":[\"LConn1\",\"In1\"]},\"type\":\"ConnectorPlacement.EquallySpacedRectSide\",\"uuid\":\"4d523b2f-3490-490d-9193-0c3e52b1c3a1\"},{\"content\":{\"connectorIds\":[\"RConn1\"],\"side\":\"RIGHT\"},\"type\":\"ConnectorPlacement.EquallySpacedRectSide\",\"uuid\":\"1543a14a-65b5-4637-8d41-6da95a6ca307\"},{\"content\":{\"side\":\"TOP\"},\"type\":\"ConnectorPlacement.EquallySpacedRectSide\",\"uuid\":\"9fff8ee8-4727-466f-977a-681c4f14cc56\"}]},\"type\":\"ConnectorPlacement.EquallySpacedConnector\",\"uuid\":\"a46df766-bf17-4bd6-a8b3-579011040ee9\"}],\"packageUris\":[\"http://schema.mathworks.com/mf0/Connector/R2020b\"],\"version\":\"1.0\"}"
  Conn2 : PMIOPort  Side=Left
  Conn1 : PMIOPort  Port=2  Side=Right
  wires:
  input0/1 -> Subsystem1/1(input0)
  connections:
  Conn2/RConn1 -- Subsystem1/RConn1
  Subsystem1/LConn1 -- Conn1/RConn1

== system VSCHVDCunitblackstart/Wind Farm/Wind Farm1/PLL & Measurements ==
  V : Inport
  Ig : Inport  Port=2
  Measurement1 : Subsystem
  Measurement2 : Subsystem
  PLL : Subsystem
  Out Bus Element : Outport  PortName=Vbus  Element=Vq
  Out Bus Element1 : Outport  PortName=Vbus  Element=Vd
  Out Bus Element2 : Outport  PortName=Vbus  Element=w
  Out Bus Element3 : Outport  PortName=Vbus  Element=Theta
  Out Bus Element4 : Outport  PortName=Vbus  Element=Vmag
  Out Bus Element5 : Outport  PortName=Vbus  Element=Id
  Out Bus Element6 : Outport  PortName=Vbus  Element=Iq
  wires:
  V/1 -> Measurement2/1(u)
  PLL/2(freq) -> Out Bus Element2/1
  PLL/5(Vq) -> Out Bus Element/1  "Vq"
  PLL/3(angle) -> Out Bus Element3/1
  PLL/4(Vd) -> Out Bus Element1/1
  Measurement2/1(Vg) -> PLL/1(abc)
  PLL/1(mag) -> Out Bus Element4/1  "Vmag"
  Measurement1/1(Ig) -> PLL/2(Ig)
  Ig/1 -> Measurement1/1(u)
  PLL/7(Iq) -> Out Bus Element6/1  "Iq"
  PLL/6(Id) -> Out Bus Element5/1  "Id"

== system VSCHVDCunitblackstart/Wind Farm/Wind Farm1/Voltage VAR Control & LVRT, FRT ==
  In Bus Element : Inport  PortName=Vbus  Element=Vmag
  In Bus Element1 : Inport  PortName=Vbus  Element=w
  Data Type Conversion : DataTypeConversion  RndMeth=Nearest  SaturateOnIntegerOverflow=off
  Delay : Delay  DelayLength=100
  Frequency RideThrough : Subsystem
  LVRT Characterstics : Subsystem
  OR : Logic  Operator=OR  IconShape=distinctive  AllPortsSameDT=off  OutDataTypeStr=boolean
  Unit Delay : UnitDelay  SampleTime=-1  HasFrameUpgradeWarning=on
  V_ref : Constant  Value=windController.vRef  SampleTime=Ts
  Voltage Control : Subsystem
  Out Bus Element : Outport  PortName=LVRT  Element=breaker
  Out Bus Element1 : Outport  PortName=LVRT  Element=iq
  Q_ref : Outport  Port=2
  wires:
  In Bus Element/1 -> LVRT Characterstics/1(Vmag), Voltage Control/1(In1)
  LVRT Characterstics/2(iq) -> Out Bus Element1/1
  V_ref/1 -> Voltage Control/2(In2)
  Voltage Control/1(Out1) -> Delay/1
  OR/1 -> Data Type Conversion/1
  LVRT Characterstics/1(Trip Signal) -> OR/1
  In Bus Element1/1 -> Frequency RideThrough/1(f)
  Data Type Conversion/1 -> Unit Delay/1
  Frequency RideThrough/1(Trip  Signal) -> OR/2
  Unit Delay/1 -> Out Bus Element/1
  Delay/1 -> Q_ref/1

== system VSCHVDCunitblackstart/Wind Farm/Wind Farm1/pitch control ==
  e : Inport
  Discrete-Time Integrator : DiscreteIntegrator  SampleTime=-1  LimitOutput=on  LowerSaturationLimit=0  ICPrevOutput=DiscIntNeverNeededParam  ICPrevScaledInput=DiscIntNeverNeededParam
  Gain1 : Gain  Gain=-5
  Gain2 : Gain  Gain=-1
  Saturation1 : Saturate  UpperLimit=inf  LowerLimit=0
  Sum1 : Sum  Inputs=|++
  Unit Delay : UnitDelay  SampleTime=-1  HasFrameUpgradeWarning=on
  pitch : Outport
  wires:
  Discrete-Time Integrator/1 -> Sum1/2
  e/1 -> Gain2/1, Gain1/1
  Saturation1/1 -> pitch/1  "pitch"
  Gain2/1 -> Discrete-Time Integrator/1
  Unit Delay/1 -> Sum1/1
  Gain1/1 -> Unit Delay/1
  Sum1/1 -> Saturation1/1

== system VSCHVDCunitblackstart/Control/Sending-end and receiving-end control/Offshore Control/Control ==
  VdcRef : Inport
  Qref : Inport  Port=2
  omega : Inport  Port=3
  theta : Inport  Port=4
  Vd : Inport  Port=5
  idg : Inport  Port=6
  iqg : Inport  Port=7
  Vdcp : Inport  Port=8
  Vdcn : Inport  Port=9
  Qmea : Inport  Port=10
  Vstart : Inport  Port=11
  Current control : Subsystem
  DC voltage and reactive power control : Subsystem
      settings: PortSchema="{\"entries\":[{\"content\":{\"sides\":[{\"content\":{\"connectorIds\":[\"In1\",\"In2\",\"In3\",\"In4\",\"In5\"]},\"type\":\"ConnectorPlacement.EquallySpacedRectSide\",\"uuid\":\"9a4f72fc-d3c2-4700-a6e4-1712802e8b48\"},{\"content\":{\"connectorIds\":[\"Out1\",\"Out2\"],\"side\":\"RIGHT\"},\"type\":\"ConnectorPlacement.EquallySpacedRectSide\",\"uuid\":\"6e2ce57a-022a-486f-97e1-9215759a688e\"},{\"content\":{\"connectorIds\":[\"In6\"],\"side\":\"TOP\"},\"type\":\"ConnectorPlacement.EquallySpacedRectSide\",\"uuid\":\"16e5a654-83a0-499b-8961-59b9a4558274\"}]},\"type\":\"ConnectorPlacement.EquallySpacedConnector\",\"uuid\":\"15ae27ba-d2ea-42ea-aa74-3055d4b53939\"}],\"packageUris\":[\"http://schema.mathworks.com/mf0/Connector/R2020b\"],\"version\":\"1.0\"}"
  NOT : Logic  Operator=NOT  IconShape=distinctive  AllPortsSameDT=off  OutDataTypeStr=boolean
  PWM generator : Subsystem
  Switch : Switch  Criteria=u2 ~= 0  SaturateOnIntegerOverflow=off  InputSameDT=off
  S : Outport
  wires:
  theta/1 -> Current control/9(theta)
  Vd/1 -> Current control/5(Vd)
  idg/1 -> Current control/3(idg)
  iqg/1 -> Current control/4(iqg)
  omega/1 -> Current control/8(omega)
  VdcRef/1 -> DC voltage and reactive power control/1(VdcRef)
  Qmea/1 -> DC voltage and reactive power control/5(Qmea)
  Vdcp/1 -> DC voltage and reactive power control/2(Vdcp), Current control/6(Vdcp)
  Vdcn/1 -> DC voltage and reactive power control/3(Vdcn), Current control/7(Vdcn)
  PWM generator/1(S) -> S/1
  Qref/1 -> DC voltage and reactive power control/4(Qref)
  DC voltage and reactive power control/1(idRef) -> Current control/1(idgRef)
  DC voltage and reactive power control/2(iqRef) -> Current control/2(iqgRef)
  Vstart/1 -> Switch/1
  NOT/1 -> DC voltage and reactive power control/6(Con)
  Current control/1(Con) -> Switch/2, NOT/1
  Switch/1 -> PWM generator/1(Vref)
  Current control/2(Vref) -> Switch/3
